simulink model "flat_data_generator"  (R2019b)
settings: Solver=FixedStepAuto  StartTime=0.0  StopTime=120  FixedStep=1/256  RelTol=1e-3
libraries: simulink x2
settings Model: Creator=Tris  LastModifiedBy=Tris

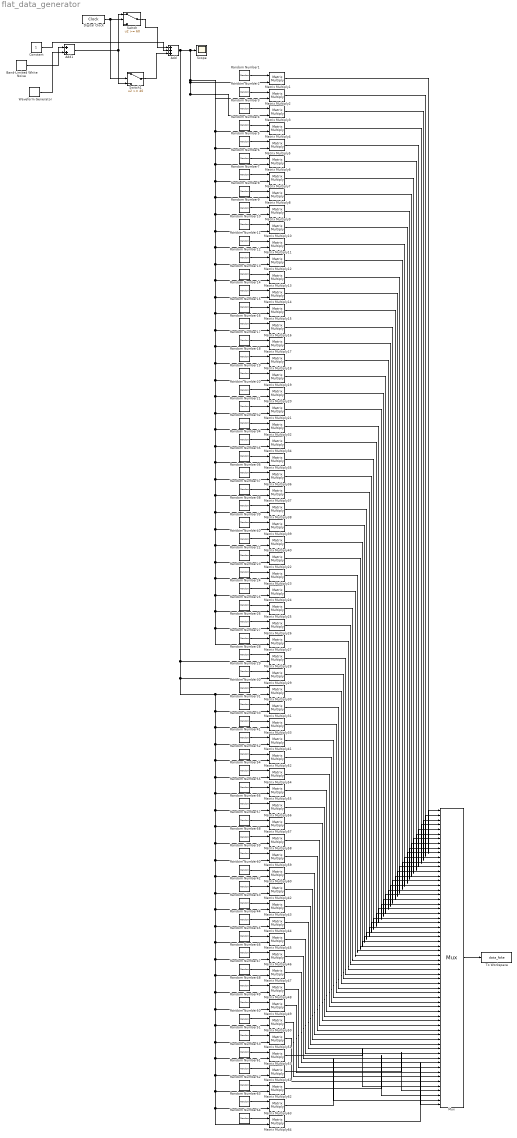
== system flat_data_generator ==
  Add : Sum  Inputs=+++
  Add1 : Sum
  Band-Limited White Noise : simulink/Sources/Band-Limited White Noise  Cov=[0.1]  Ts=1/256  seed=[23341]
  Constant : Constant
  Digital Clock : DigitalClock  SampleTime=1/256
  Matrix Multiply{1..64} (64 alike) : Product  Multiplication=Matrix(*)
  Mux : Mux  Inputs=64
  Random Number1 : RandomNumber  Mean=1  Variance=0.2  Seed=1  SampleTime=1/256
  Random Number10 : RandomNumber  Mean=1  Variance=0.2  Seed=1  SampleTime=1/256
  Random Number11 : RandomNumber  Mean=1  Variance=0.2  Seed=11  SampleTime=1/256
  Random Number12 : RandomNumber  Mean=1  Variance=0.2  Seed=12  SampleTime=1/256
  Random Number13 : RandomNumber  Mean=1  Variance=0.2  Seed=13  SampleTime=1/256
  Random Number14 : RandomNumber  Mean=1  Variance=0.2  Seed=14  SampleTime=1/256
  Random Number15 : RandomNumber  Mean=1  Variance=0.2  Seed=15  SampleTime=1/256
  Random Number16 : RandomNumber  Mean=1  Variance=0.2  Seed=16  SampleTime=1/256
  Random Number17 : RandomNumber  Mean=1  Variance=0.2  Seed=17  SampleTime=1/256
  Random Number18 : RandomNumber  Mean=1  Variance=0.2  Seed=18  SampleTime=1/256
  Random Number19 : RandomNumber  Mean=1  Variance=0.2  Seed=19  SampleTime=1/256
  Random Number2 : RandomNumber  Mean=1  Variance=0.2  Seed=1  SampleTime=1/256
  Random Number20 : RandomNumber  Mean=1  Variance=0.2  Seed=20  SampleTime=1/256
  Random Number21 : RandomNumber  Mean=1  Variance=0.2  Seed=21  SampleTime=1/256
  Random Number22 : RandomNumber  Mean=1  Variance=0.2  Seed=30  SampleTime=1/256
  Random Number23 : RandomNumber  Mean=1  Variance=0.2  Seed=31  SampleTime=1/256
  Random Number24 : RandomNumber  Mean=1  Variance=0.2  Seed=32  SampleTime=1/256
  Random Number25 : RandomNumber  Mean=1  Variance=0.2  Seed=33  SampleTime=1/256
  Random Number26 : RandomNumber  Mean=1  Variance=0.2  Seed=34  SampleTime=1/256
  Random Number27 : RandomNumber  Mean=1  Variance=0.2  Seed=35  SampleTime=1/256
  Random Number28 : RandomNumber  Mean=1  Variance=0.2  Seed=36  SampleTime=1/256
  Random Number29 : RandomNumber  Mean=1  Variance=0.2  Seed=37  SampleTime=1/256
  Random Number3 : RandomNumber  Mean=1  Variance=0.2  Seed=4  SampleTime=1/256
  Random Number30 : RandomNumber  Mean=1  Variance=0.2  Seed=38  SampleTime=1/256
  Random Number31 : RandomNumber  Mean=1  Variance=0.2  Seed=39  SampleTime=1/256
  Random Number32 : RandomNumber  Mean=1  Variance=0.2  Seed=22  SampleTime=1/256
  Random Number33 : RandomNumber  Mean=1  Variance=0.2  Seed=40  SampleTime=1/256
  Random Number34 : RandomNumber  Mean=1  Variance=0.2  Seed=23  SampleTime=1/256
  Random Number35 : RandomNumber  Mean=1  Variance=0.2  Seed=24  SampleTime=1/256
  Random Number36 : RandomNumber  Mean=1  Variance=0.2  Seed=25  SampleTime=1/256
  Random Number37 : RandomNumber  Mean=1  Variance=0.2  Seed=26  SampleTime=1/256
  Random Number38 : RandomNumber  Mean=1  Variance=0.2  Seed=27  SampleTime=1/256
  Random Number39 : RandomNumber  Mean=1  Variance=0.2  Seed=28  SampleTime=1/256
  Random Number4 : RandomNumber  Mean=1  Variance=0.2  Seed=5  SampleTime=1/256
  Random Number40 : RandomNumber  Mean=1  Variance=0.2  Seed=29  SampleTime=1/256
  Random Number41 : RandomNumber  Mean=1  Variance=0.2  Seed=41  SampleTime=1/256
  Random Number42 : RandomNumber  Mean=1  Variance=0.2  Seed=50  SampleTime=1/256
  Random Number43 : RandomNumber  Mean=1  Variance=0.2  Seed=51  SampleTime=1/256
  Random Number44 : RandomNumber  Mean=1  Variance=0.2  Seed=52  SampleTime=1/256
  Random Number45 : RandomNumber  Mean=1  Variance=0.2  Seed=53  SampleTime=1/256
  Random Number46 : RandomNumber  Mean=1  Variance=0.2  Seed=54  SampleTime=1/256
  Random Number47 : RandomNumber  Mean=1  Variance=0.2  Seed=55  SampleTime=1/256
  Random Number48 : RandomNumber  Mean=1  Variance=0.2  Seed=56  SampleTime=1/256
  Random Number49 : RandomNumber  Mean=1  Variance=0.2  Seed=57  SampleTime=1/256
  Random Number5 : RandomNumber  Mean=1  Variance=0.2  Seed=6  SampleTime=1/256
  Random Number50 : RandomNumber  Mean=1  Variance=0.2  Seed=58  SampleTime=1/256
  Random Number51 : RandomNumber  Mean=1  Variance=0.2  Seed=59  SampleTime=1/256
  Random Number52 : RandomNumber  Mean=1  Variance=0.2  Seed=42  SampleTime=1/256
  Random Number53 : RandomNumber  Mean=1  Variance=0.2  Seed=60  SampleTime=1/256
  Random Number54 : RandomNumber  Mean=1  Variance=0.2  Seed=43  SampleTime=1/256
  Random Number55 : RandomNumber  Mean=1  Variance=0.2  Seed=44  SampleTime=1/256
  Random Number56 : RandomNumber  Mean=1  Variance=0.2  Seed=45  SampleTime=1/256
  Random Number57 : RandomNumber  Mean=1  Variance=0.2  Seed=46  SampleTime=1/256
  Random Number58 : RandomNumber  Mean=1  Variance=0.2  Seed=47  SampleTime=1/256
  Random Number59 : RandomNumber  Mean=1  Variance=0.2  Seed=48  SampleTime=1/256
  Random Number6 : RandomNumber  Mean=1  Variance=0.2  Seed=7  SampleTime=1/256
  Random Number60 : RandomNumber  Mean=1  Variance=0.2  Seed=49  SampleTime=1/256
  Random Number61 : RandomNumber  Mean=1  Variance=0.2  Seed=61  SampleTime=1/256
  Random Number62 : RandomNumber  Mean=1  Variance=0.2  Seed=62  SampleTime=1/256
  Random Number63 : RandomNumber  Mean=1  Variance=0.2  Seed=63  SampleTime=1/256
  Random Number64 : RandomNumber  Mean=1  Variance=0.2  Seed=64  SampleTime=1/256
  Random Number7 : RandomNumber  Mean=1  Variance=0.2  Seed=8  SampleTime=1/256
  Random Number8 : RandomNumber  Mean=1  Variance=0.2  Seed=9  SampleTime=1/256
  Random Number9 : RandomNumber  Mean=1  Variance=0.2  Seed=10  SampleTime=1/256
  Scope : Scope
  Switch : Switch  Threshold=60
  Switch1 : Switch  Threshold=40
  To Workspace : ToWorkspace  VariableName=data_fake  SaveFormat=Timeseries  SampleTime=-1
  Waveform Generator : simulink/Sources/Waveform Generator  OutMin=[]  OutMax=[]  OutDataTypeStr=double  SelectedSignal=1  Signals=sin(2,2,0)#sin(2,15,0)#sin(2,30,0)#sin(2,20,0)  BlockNames=MultiportSwitch_9a07a450d4bd44b#MultiportSwitch_a51acfa1090d4b1#MultiportSwitch_bf0259e5e1ce4d7#MultiportSwitch_60f36bc4c477490  SampleTime=1/256
      settings: SourceProductName=Simulink
  wires:
  Switch/1 -> Add/1
  Digital Clock/1 -> Switch1/2, Switch/2
  Switch1/1 -> Add/3
  Constant/1 -> Add/2
  Add1/1 -> Switch1/3, Switch/1
  Waveform Generator/1 -> Add1/2
  Random Number1/1 -> Matrix Multiply1/1
  Random Number2/1 -> Matrix Multiply2/1
  Random Number3/1 -> Matrix Multiply3/1
  Random Number4/1 -> Matrix Multiply4/1
  Random Number6/1 -> Matrix Multiply6/1
  Random Number5/1 -> Matrix Multiply5/1
  Random Number7/1 -> Matrix Multiply7/1
  Random Number8/1 -> Matrix Multiply8/1
  Random Number10/1 -> Matrix Multiply10/1
  Random Number9/1 -> Matrix Multiply9/1
  Random Number11/1 -> Matrix Multiply11/1
  Random Number12/1 -> Matrix Multiply12/1
  Random Number14/1 -> Matrix Multiply14/1
  Random Number13/1 -> Matrix Multiply13/1
  Random Number15/1 -> Matrix Multiply15/1
  Random Number16/1 -> Matrix Multiply16/1
  Random Number18/1 -> Matrix Multiply18/1
  Random Number17/1 -> Matrix Multiply17/1
  Random Number19/1 -> Matrix Multiply19/1
  Random Number20/1 -> Matrix Multiply20/1
  Random Number28/1 -> Matrix Multiply28/1
  Random Number25/1 -> Matrix Multiply25/1
  Random Number27/1 -> Matrix Multiply27/1
  Random Number24/1 -> Matrix Multiply24/1
  Random Number22/1 -> Matrix Multiply22/1
  Random Number40/1 -> Matrix Multiply40/1
  Random Number26/1 -> Matrix Multiply26/1
  Random Number23/1 -> Matrix Multiply23/1
  Random Number32/1 -> Matrix Multiply32/1
  Random Number30/1 -> Matrix Multiply30/1
  Random Number34/1 -> Matrix Multiply34/1
  Random Number31/1 -> Matrix Multiply31/1
  Random Number29/1 -> Matrix Multiply29/1
  Random Number33/1 -> Matrix Multiply33/1
  Random Number39/1 -> Matrix Multiply39/1
  Random Number38/1 -> Matrix Multiply38/1
  Random Number21/1 -> Matrix Multiply21/1
  Random Number36/1 -> Matrix Multiply36/1
  Random Number35/1 -> Matrix Multiply35/1
  Random Number37/1 -> Matrix Multiply37/1
  Random Number48/1 -> Matrix Multiply48/1
  Random Number45/1 -> Matrix Multiply45/1
  Random Number47/1 -> Matrix Multiply47/1
  Random Number44/1 -> Matrix Multiply44/1
  Random Number42/1 -> Matrix Multiply42/1
  Random Number60/1 -> Matrix Multiply60/1
  Random Number46/1 -> Matrix Multiply46/1
  Random Number43/1 -> Matrix Multiply43/1
  Random Number52/1 -> Matrix Multiply52/1
  Random Number50/1 -> Matrix Multiply50/1
  Random Number54/1 -> Matrix Multiply54/1
  Random Number51/1 -> Matrix Multiply51/1
  Random Number49/1 -> Matrix Multiply49/1
  Random Number53/1 -> Matrix Multiply53/1
  Random Number59/1 -> Matrix Multiply59/1
  Random Number58/1 -> Matrix Multiply58/1
  Random Number41/1 -> Matrix Multiply41/1
  Random Number56/1 -> Matrix Multiply56/1
  Random Number55/1 -> Matrix Multiply55/1
  Random Number57/1 -> Matrix Multiply57/1
  Random Number61/1 -> Matrix Multiply61/1
  Random Number62/1 -> Matrix Multiply62/1
  Random Number63/1 -> Matrix Multiply63/1
  Matrix Multiply1/1 -> Mux/1
  Matrix Multiply2/1 -> Mux/2
  Matrix Multiply3/1 -> Mux/3
  Matrix Multiply4/1 -> Mux/4
  Matrix Multiply5/1 -> Mux/5
  Matrix Multiply6/1 -> Mux/6
  Matrix Multiply7/1 -> Mux/7
  Matrix Multiply8/1 -> Mux/8
  Matrix Multiply9/1 -> Mux/9
  Matrix Multiply10/1 -> Mux/10
  Matrix Multiply11/1 -> Mux/11
  Matrix Multiply12/1 -> Mux/12
  Matrix Multiply13/1 -> Mux/13
  Matrix Multiply14/1 -> Mux/14
  Matrix Multiply15/1 -> Mux/15
  Matrix Multiply16/1 -> Mux/16
  Matrix Multiply17/1 -> Mux/17
  Matrix Multiply18/1 -> Mux/18
  Matrix Multiply19/1 -> Mux/19
  Matrix Multiply20/1 -> Mux/20
  Matrix Multiply21/1 -> Mux/21
  Matrix Multiply32/1 -> Mux/22
  Matrix Multiply34/1 -> Mux/23
  Matrix Multiply35/1 -> Mux/24
  Matrix Multiply36/1 -> Mux/25
  Matrix Multiply37/1 -> Mux/26
  Matrix Multiply38/1 -> Mux/27
  Matrix Multiply39/1 -> Mux/28
  Matrix Multiply40/1 -> Mux/29
  Matrix Multiply22/1 -> Mux/30
  Matrix Multiply23/1 -> Mux/31
  Matrix Multiply24/1 -> Mux/32
  Matrix Multiply25/1 -> Mux/33
  Matrix Multiply26/1 -> Mux/34
  Matrix Multiply27/1 -> Mux/35
  Matrix Multiply28/1 -> Mux/36
  Matrix Multiply29/1 -> Mux/37
  Matrix Multiply30/1 -> Mux/38
  Matrix Multiply31/1 -> Mux/39
  Matrix Multiply33/1 -> Mux/40
  Matrix Multiply41/1 -> Mux/41
  Matrix Multiply52/1 -> Mux/42
  Matrix Multiply54/1 -> Mux/43
  Matrix Multiply55/1 -> Mux/44
  Matrix Multiply56/1 -> Mux/45
  Matrix Multiply57/1 -> Mux/46
  Matrix Multiply58/1 -> Mux/47
  Matrix Multiply59/1 -> Mux/48
  Matrix Multiply60/1 -> Mux/49
  Matrix Multiply42/1 -> Mux/50
  Matrix Multiply43/1 -> Mux/51
  Matrix Multiply44/1 -> Mux/52
  Matrix Multiply45/1 -> Mux/53
  Matrix Multiply46/1 -> Mux/54
  Matrix Multiply47/1 -> Mux/55
  Matrix Multiply48/1 -> Mux/56
  Matrix Multiply49/1 -> Mux/57
  Matrix Multiply50/1 -> Mux/58
  Matrix Multiply51/1 -> Mux/59
  Matrix Multiply53/1 -> Mux/60
  Matrix Multiply61/1 -> Mux/61
  Matrix Multiply62/1 -> Mux/62
  Matrix Multiply63/1 -> Mux/63
  Add/1 -> Matrix Multiply42/2, Matrix Multiply64/2, Matrix Multiply63/2, Matrix Multiply62/2, Matrix Multiply61/2, Matrix Multiply53/2, Matrix Multiply51/2, Matrix Multiply50/2, Matrix Multiply49/2, Matrix Multiply48/2, Matrix Multiply47/2, Matrix Multiply46/2, Matrix Multiply45/2, Matrix Multiply44/2, Matrix Multiply43/2, Matrix Multiply60/2, Matrix Multiply59/2, Matrix Multiply58/2, Matrix Multiply57/2, Matrix Multiply56/2, Matrix Multiply55/2, Matrix Multiply54/2, Matrix Multiply52/2, Matrix Multiply41/2, Matrix Multiply33/2, Matrix Multiply31/2, Matrix Multiply30/2, Matrix Multiply29/2, Matrix Multiply28/2, Matrix Multiply2/2, Matrix Multiply27/2, Matrix Multiply26/2, Matrix Multiply25/2, Matrix Multiply24/2, Matrix Multiply23/2, Matrix Multiply22/2, Matrix Multiply40/2, Matrix Multiply39/2, Matrix Multiply38/2, Matrix Multiply37/2, Matrix Multiply36/2, Matrix Multiply35/2, Matrix Multiply34/2, Matrix Multiply32/2, Matrix Multiply21/2, Matrix Multiply20/2, Matrix Multiply19/2, Matrix Multiply18/2, Matrix Multiply17/2, Matrix Multiply16/2, Matrix Multiply15/2, Matrix Multiply14/2, Matrix Multiply13/2, Matrix Multiply12/2, Matrix Multiply11/2, Matrix Multiply10/2, Matrix Multiply9/2, Matrix Multiply8/2, Matrix Multiply7/2, Matrix Multiply6/2, Matrix Multiply5/2, Matrix Multiply4/2, Matrix Multiply3/2, Matrix Multiply1/2, Scope/1
  Random Number64/1 -> Matrix Multiply64/1
  Matrix Multiply64/1 -> Mux/64
  Mux/1 -> To Workspace/1
  Band-Limited White Noise/1 -> Add1/1
